simulink model "JAndrews_Test"  (R2019b)
settings: Solver=VariableStepAuto  StartTime=0.0  StopTime=10.0  RelTol=1e-3
settings Model: Creator=ng21251  LastModifiedBy=ng21251

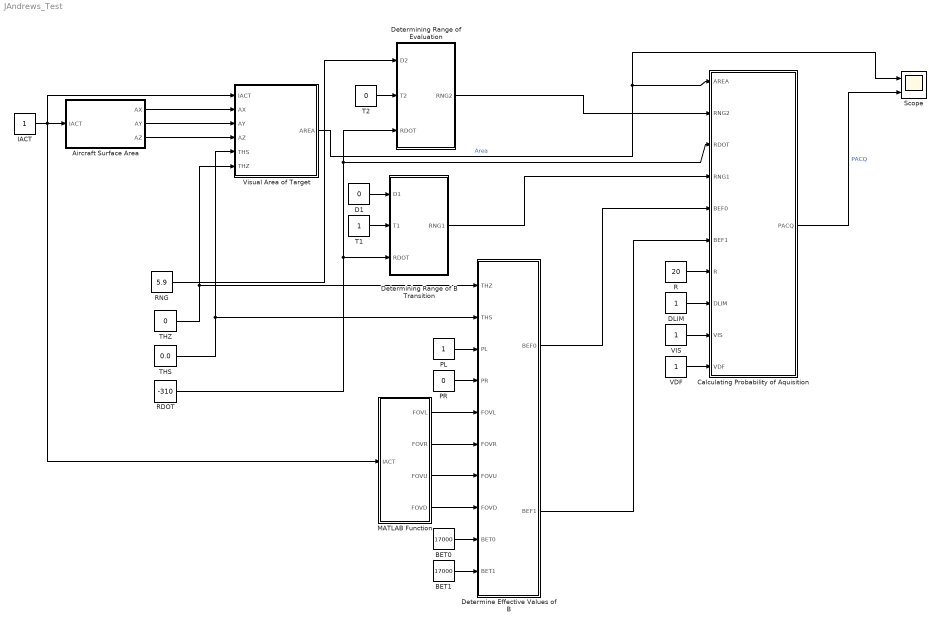
== system JAndrews_Test ==
  Aircraft Surface Area : MATLAB Function  TreatAsAtomicUnit=on
  BET0 : Constant  Value=17000
  BET1 : Constant  Value=17000
  Calculating Probability of Aquisition : MATLAB Function  TreatAsAtomicUnit=on
  D1 : Constant  Value=0
  DLIM : Constant
  Determine Effective Values of B : MATLAB Function  TreatAsAtomicUnit=on
  Determining Range of B Transition : MATLAB Function  TreatAsAtomicUnit=on
  Determining Range of Evaluation : MATLAB Function  TreatAsAtomicUnit=on
  "IACT " : Constant
  MATLAB Function : MATLAB Function  TreatAsAtomicUnit=on
  PL : Constant
  PR : Constant  Value=0
  R : Constant  Value=20
  "RDOT " : Constant  Value=-310
  "RNG " : Constant  Value=5.9
  Scope : Scope  NumInputPorts=2
  T1 : Constant
  T2 : Constant  Value=0
  THS : Constant  Value=0.0
  THZ : Constant  Value=0
  "VDF " : Constant
  VIS : Constant
  Visual Area of Target : MATLAB Function  TreatAsAtomicUnit=on
  wires:
  MATLAB Function/2(FOVR) -> Determine Effective Values of B/6(FOVR)
  Determining Range of Evaluation/1(RNG2) -> Calculating Probability of Aquisition/2(RNG2)
  "IACT "/1 -> Visual Area of Target/1(IACT), MATLAB Function/1(IACT), Aircraft Surface Area/1(IACT)
  Determine Effective Values of B/1(BEF0) -> Calculating Probability of Aquisition/5(BEF0)
  "RNG "/1 -> Determining Range of Evaluation/1(D2)
  Visual Area of Target/1(AREA) -> Scope/1, Calculating Probability of Aquisition/1(AREA)  "Area"
  R/1 -> Calculating Probability of Aquisition/7(R)
  DLIM/1 -> Calculating Probability of Aquisition/8(DLIM)
  Determine Effective Values of B/2(BEF1) -> Calculating Probability of Aquisition/6(BEF1)
  Aircraft Surface Area/2(AY) -> Visual Area of Target/3(AY)
  T2/1 -> Determining Range of Evaluation/2(T2)
  D1/1 -> Determining Range of B Transition/1(D1)
  Aircraft Surface Area/1(AX) -> Visual Area of Target/2(AX)
  Determining Range of B Transition/1(RNG1) -> Calculating Probability of Aquisition/4(RNG1)
  PL/1 -> Determine Effective Values of B/3(PL)
  MATLAB Function/1(FOVL) -> Determine Effective Values of B/5(FOVL)
  Aircraft Surface Area/3(AZ) -> Visual Area of Target/4(AZ)
  THS/1 -> Determine Effective Values of B/2(THS), Visual Area of Target/5(THS)
  PR/1 -> Determine Effective Values of B/4(PR)
  T1/1 -> Determining Range of B Transition/2(T1)
  "RDOT "/1 -> Determining Range of B Transition/3(RDOT), Determining Range of Evaluation/3(RDOT), Calculating Probability of Aquisition/3(RDOT)
  Calculating Probability of Aquisition/1(PACQ) -> Scope/2  "PACQ"
  THZ/1 -> Determine Effective Values of B/1(THZ), Visual Area of Target/6(THZ)
  BET0/1 -> Determine Effective Values of B/9(BET0)
  BET1/1 -> Determine Effective Values of B/10(BET1)
  MATLAB Function/4(FOVD) -> Determine Effective Values of B/8(FOVD)
  MATLAB Function/3(FOVU) -> Determine Effective Values of B/7(FOVU)
  "VDF "/1 -> Calculating Probability of Aquisition/10(VDF)
  VIS/1 -> Calculating Probability of Aquisition/9(VIS)

== matlab function JAndrews_Test/Calculating Probability of Aquisition ==
  data: AREA input; PACQ output; RNG2 input; RDOT input; RNG1 input; BEF0 input; BEF1 input; R input; DLIM input; VIS input; VDF input
function PACQ = JAndrews_Mod_7(AREA, RNG2, RDOT, RNG1, BEF0, BEF1, R, DLIM, VIS, VDF)
% Input variable defintions
% No, symbol, name, value, definition
% 7.  R,  R,    20. nmi,                  visual range
% 8.  d,  DLIM, 1 arc-min,                Resolution limit of human eye.
% 17. r., RDOT, 380 kt*,                  Range rate of target aircraft
% 21. A,  AREA, 35 sq.ft.*,               Final visual area of target.
% 24. R1, RNG1, 3.78 nmi*,                Range at which B transition occurs.
% 25. R2, RNG2, 1.27 nmi*,                Range at which PACQ is evaluated.
% 26. B0, BEF0, 17000* per steradian-sec, Effective value of B before transition.
% 27. B1, BEF1, 17000* per steradian-sec, Effective value of B after transition.
% 28. P, PACQ,  -                         Probability of visual aquisition
% *=value that is computed when all 16 input variables have nominal value.
 
 
% 4.2.7 Module 7: timputing the Wmulative Probability of kquiaition
% M
% Module 7 ia the final module that actually computes the probability of
% visual acquisition, PACQ. It requires 8 inputa aa ahom in Fig. 4.1.
% Module 7 aaaumes that the acquisition rate drops immediately to zero when
% the target ia beyond a range, RLIM, corresponding to the resolution limit of
% the human eye. RLIM ia defined aa follows: First, DL~, WA, and RDOT are
% used to compute the range at which the solid angle subtended by the target
% equals that of a circle with diameter DL~. This range ia given by the
% formula
% 1.1284*SQRT(AREA)/DLIM
% where DL~ ia in radiana. Then, if this range is greater than R, the visual
% range, it is reduced to R. The net result ia
% RLIM = ndnimum [1.1284*SQRT(A~A)/DLIM, R]
% A more aophieticated model for MIM could be constructed, but in meet
% analyaea, only a tiny fraction of the opportunity for visual acquieition
% occurs before the target ie well within visual range and well above the
% resolution threshold. Wnce, the detaile of the model in this regard are
% normally of little consequence.
% Note that if RLIM ia less than RNGl, then % till already have
% transitioned to BET1 before the target is close enough to be seen. b this
% caae, the value of BETO has no affect upon the calculation.
 
%Range limit = the minimum of either the human eye distinguishing target size or visual range
RLIM = min([ 1.1284 * (AREA)^0.5 / DLIM, R]);

%if the eval range is beyond these two - cannot detect
if RNG2 > RLIM 
    PACQ=0;
    
else
    
%else
    rng3=intcalcforce(AREA,RNG2,RDOT);
    pacq_3= BEF0*(rng3)*VIS*VDF;
    PACQ=1.0-exp(-pacq_3);

end


function x_e = intcalcforce(A,B,C)
T2=0:0.0001:1;

tmp=(A./(B+C*T2).^2).* exp(-2.996 * (B+C*T2));
x_e=sum(tmp*0.0001)*((numel(T2)-1)/numel(T2));

== matlab function JAndrews_Test/Visual Area of Target ==
  data: IACT input; AX input; AREA output; AY input; AZ input; THS input; THZ input
function AREA = JAndrews_Mod_3(IACT,AX, AY, AZ, THS, THZ)
% Input variable defintions
% No, symbol, name, value, definition
% 18. Ax, AX,   35 sq.ft.*,               Head-on visual area of target.
% 19. Ay, AY,   85 sq.ft.*,               Broadside visual area of target.
% 20. Az, AZ,   260 sq.ft.*,              Topside visual area of target.
% 21. A,  AREA, 35 sq.ft.*,               Final visual area of target.
% 22. 0T, TH1,  0 deg*,                   Bearing of target aircraft as seen from subject aircraft.
% 23. 0S, TH2,  0 deg*,                   Bearing of subject aircraft as seen from target aircraft.
% 24. R1, RNG1, 3.78 nmi*,                Range at which B transition occurs.
% 25. R2, RNG2, 1.27 nmi*,                Range at which PACQ is evaluated.
% 26. B0, BEF0, 17000* per steradian-sec, Effective value of B before transition.
% 27. B1, BEF1, 17000* per steradian-sec, Effective value of B after transition.
% 28. P, PACQ,  -                         Probability of visual aquisition
% *=value that is computed when all 16 input variables have nominal value.



%%-------MODULE 3---------
% 4.2.3 Module 3: Computing the Visual Area of the Target
% The visual area of the target ie computed by projecting the principal
% visual areas AX and AY onto a plane that is normal to the linemf-sfght
% between the two aircraft. ~is plane is at an angle ~ with respect to the
% Y-Z plane for the target aircraft. h approximate correction for shielding ie
% applied by assudng that the actual visual area is the largest of the
% projectione of M and AY plus one+hird of the smallest projection (see
% Mference 2). ~is approximation is errorless when the aircraft ie viewed
% along one of the principal axas. Because Mdule 3 assumes that the
% line-f =ight lies tithin the X-Y plane, the topside area, AZ, ie not allowed
% to centribute to the target visual area. This ia normally a good assumption,
% but can result in underestimation of the visual area if the pitch angle of the
% aircraft is large. U is defined in the module to allow for future exteneion
% of the software.



if IACT>7
% aclist=[...
% 'a10 ';'a109';'a306';'a310';'a318';'a319';'a320';'a321';'a332';'a333';'a342';
% 'a343';'a345';'a346';'a6  ';'aa5 ';'aest';'as32';'as50';'as55';'as65';'astr';'at72';
% 'b06 ';'b190';'b2  ';'b200';'b206';'b222';'b350';'b400';'b412';'b427';'b461';'b462';
% 'b52 ';'b703';'b712';'b721';'b722';'b731';'b732';'b733';'b734';'b735';'b737';'b738';
% 'b743';'b744';'b752';'b753';'b762';'b763';'b772';'b773';'be18';'be20';'be35';'be40';
% 'be50';'be56';'be58';'be60';'be70';'be90';'be99';'bk17';'c130';'c141';'c152';'c17 ';
% 'c172';'c177';'c182';'c185';'c206';'c208';'c210';'c212';'c310';'c402';'c5  ';'c500';
% 'c680';'c750';'cl60';'col3';'crj1';'crj2';'crj7';'crj9';'d328';'dc10';'dc3 ';'dc91';
% 'dc93';'dc95';'dh8a';'dh8b';'dh8c';'dh8d';'e110';'e121';'e135';'e145';'e170';'e190';
% 'e2  ';'e45x';'e767';'ec20';'ec35';'ec45';'f100';'f14 ';'f15 ';'f16 ';'f18 ';'f22 ';
% 'f2th';'f900';'fa10';'fa50';'galx';'glex';'glf4';'glf5';'h25b';'h47 ';'h500';'h53s';
% 'h60 ';'h64 ';'huco';'js31';'k35e';'k35r';'lj31';'lj35';'lj45';'lj60';'m20p';'md11';
% 'md60';'md81';'md82';'md83';'md88';'mi2 ';'mi24';'mi28';'mu2 ';'p28a';'p3  ';'pa11';
% 'pa22';'pa23';'pa31';'pa32';'pa44';'pa46';'pc12';'r22 ';'rq1 ';'rq4a';'s360';'s65c';
% 'sf34';'sh33';'sr20';'sr71';'sw4 ';'u2  ';'uh1 ';'v22 ';'vc10';'ww24'];
AREA_S=[     0   -90   414
    15   -90   591
    30   -90   601
    45   -90   588
    60   -90   591
    75   -90   589
    90   -90   414
   105   -90   596
   120   -90   602
   135   -90   588
   150   -90   591
   165   -90   591
   180   -90   416
   195   -90   591
   210   -90   601
   225   -90   588
   240   -90   596
   255   -90   589
   270   -90   416
   285   -90   601
   300   -90   601
   315   -90   589
   330   -90   591
   345   -90   589
   360   -90   414
     0   -75   392
    15   -75   392
    30   -75   388
    45   -75   407
    60   -75   413
    75   -75   566
    90   -75   485
   105   -75   444
   120   -75   444
   135   -75   434
   150   -75   469
   165   -75   546
   180   -75   546
   195   -75   543
   210   -75   428
   225   -75   461
   240   -75   472
   255   -75   472
   270   -75   468
   285   -75   478
   300   -75   407
   315   -75   401
   330   -75   382
   345   -75   380
   360   -75   392
     0   -60   339
    15   -60   360
    30   -60   430
    45   -60   441
    60   -60   481
    75   -60   540
    90   -60   540
   105   -60   463
   120   -60   448
   135   -60   517
   150   -60   511
   165   -60   506
   180   -60   499
   195   -60   494
   210   -60   500
   225   -60   427
   240   -60   450
   255   -60   440
   270   -60   461
   285   -60   535
   300   -60   481
   315   -60   441
   330   -60   426
   345   -60   358
   360   -60   339
     0   -45   271
    15   -45   353
    30   -45   374
    45   -45   392
    60   -45   387
    75   -45   359
    90   -45   356
   105   -45   376
   120   -45   431
   135   -45   437
   150   -45   431
   165   -45   412
   180   -45   407
   195   -45   416
   210   -45   414
   225   -45   442
   240   -45   375
   255   -45   386
   270   -45   329
   285   -45   344
   300   -45   336
   315   -45   380
   330   -45   376
   345   -45   352
   360   -45   271
     0   -30   333
    15   -30   345
    30   -30   349
    45   -30   366
    60   -30   348
    75   -30   292
    90   -30   312
   105   -30   290
   120   -30   356
   135   -30   343
   150   -30   327
   165   -30   327
   180   -30   297
   195   -30   323
   210   -30   337
   225   -30   345
   240   -30   357
   255   -30   300
   270   -30   294
   285   -30   280
   300   -30   336
   315   -30   363
   330   -30   357
   345   -30   344
   360   -30   333
     0   -15   229
    15   -15   247
    30   -15   259
    45   -15   243
    60   -15   315
    75   -15   305
    90   -15   275
   105   -15   314
   120   -15   290
   135   -15   253
   150   -15   216
   165   -15   229
   180   -15   189
   195   -15   250
   210   -15   216
   225   -15   250
   240   -15   289
   255   -15   314
   270   -15   278
   285   -15   276
   300   -15   314
   315   -15   237
   330   -15   244
   345   -15   248
   360   -15   229
     0     0   125
    15     0   180
    30     0   206
    45     0   208
    60     0   264
    75     0   289
    90     0   288
   105     0   280
   120     0   265
   135     0   208
   150     0   202
   165     0   182
   180     0   125
   195     0   180
   210     0   206
   225     0   208
   240     0   264
   255     0   289
   270     0   288
   285     0   280
   300     0   265
   315     0   208
   330     0   202
   345     0   182
   360     0   125
     0    15   192
    15    15   250
    30    15   216
    45    15   250
    60    15   289
    75    15   314
    90    15   278
   105    15   276
   120    15   314
   135    15   237
   150    15   244
   165    15   248
   180    15   229
   195    15   247
   210    15   259
   225    15   243
   240    15   315
   255    15   305
   270    15   275
   285    15   314
   300    15   290
   315    15   253
   330    15   216
   345    15   229
   360    15   192
     0    30   299
    15    30   323
    30    30   337
    45    30   345
    60    30   357
    75    30   300
    90    30   294
   105    30   280
   120    30   336
   135    30   363
   150    30   357
   165    30   344
   180    30   333
   195    30   345
   210    30   349
   225    30   366
   240    30   348
   255    30   292
   270    30   312
   285    30   290
   300    30   356
   315    30   343
   330    30   327
   345    30   327
   360    30   299
     0    45   405
    15    45   416
    30    45   414
    45    45   442
    60    45   375
    75    45   386
    90    45   329
   105    45   344
   120    45   336
   135    45   380
   150    45   376
   165    45   352
   180    45   271
   195    45   353
   210    45   374
   225    45   392
   240    45   387
   255    45   359
   270    45   356
   285    45   376
   300    45   431
   315    45   437
   330    45   431
   345    45   412
   360    45   405
     0    60   496
    15    60   494
    30    60   500
    45    60   427
    60    60   450
    75    60   440
    90    60   461
   105    60   535
   120    60   481
   135    60   441
   150    60   426
   165    60   358
   180    60   339
   195    60   360
   210    60   430
   225    60   441
   240    60   481
   255    60   540
   270    60   540
   285    60   463
   300    60   448
   315    60   517
   330    60   511
   345    60   506
   360    60   496
     0    75   546
    15    75   543
    30    75   428
    45    75   461
    60    75   472
    75    75   472
    90    75   468
   105    75   478
   120    75   407
   135    75   401
   150    75   382
   165    75   375
   180    75   396
   195    75   399
   210    75   388
   225    75   407
   240    75   413
   255    75   566
   270    75   485
   285    75   444
   300    75   444
   315    75   434
   330    75   469
   345    75   546
   360    75   546
     0    90   414
    15    90   596
    30    90   601
    45    90   588
    60    90   596
    75    90   591
    90    90   416
   105    90   591
   120    90   601
   135    90   589
   150    90   596
   165    90   591
   180    90   414
   195    90   596
   210    90   601
   225    90   589
   240    90   591
   255    90   589
   270    90   414
   285    90   601
   300    90   602
   315    90   589
   330    90   596
   345    90   589
   360    90   414];

    THSdiff=abs(AREA_S(:,1)-THS);
    THZdiff=abs(AREA_S(:,2)-THZ);
    mTHS=min(THSdiff);
    mTHZ=min(THZdiff);
    
    %find the closest angle combination
    indx=ismember(THSdiff,mTHS)&ismember(THZdiff,mTHZ);
    
    %make a list of indicies
    %find the incidices that are the closest
    %take the first instance only
    indxnum=1:numel(indx);
    indxnum=indxnum(indx>0);
    indxnum=indxnum(1);
    
    %area = first smallest index - convert to nm^2
    AREA=AREA_S(indxnum,3)/6076.115486;
    
    
else

XArea = abs(cos(deg2rad(THS))) * abs(cos(deg2rad(THZ))) * AX;
YArea = abs(sin(deg2rad(THS))) * abs(cos(deg2rad(THZ))) * AY;

ZArea = abs(sin(deg2rad(THZ))) * AZ;



AREA = XArea + YArea + ZArea;
AREA=AREA/6076.115486;
end

== matlab function JAndrews_Test/Aircraft Surface Area ==
  data: IACT input; AX output; AY output; AZ output
function [AX, AY, AZ] = JAndrews_Mod_1(IACT)

% Input variable defintions
% No, symbol, name, value, definition
% 1.  - , BET0, 17000 per steradian-sec,  single pilot B values before transition
% 2.  - , BET1, 17000 per steradian-sec,  Single-pilot B value after transition
% 3.  t1, T1,   180 sec,                  modified tau time for B transition (time to closest approach)
% 4.  t2, T2,   12 sec,                   modified tau time for evaluation of PACQ (time to closest approach)
% 5.  D1, D1,   0. nmi,                   modified tau range parameter for B transition.
% 6.  D2, D2,   0. nmi,                   modified tau range parameter for PACQ evaluation
% 7.  R,  R,    20. nmi,                  visual range
% 8.  d,  DLIM, 1 arc-min,                Resolution limit of human eye.
% 9.  V1, VSUB1,180 kt,                   airspeed of subject aircraft.
% 10. V2, VSUB2,130 kt,                   airspeed of target aircraft.
% 11. - , IACT, 1,                        aircraft type for target aircraft (see table)
% 12. X,  XANG, 180. deg,                 Crossing angle (relative heading)
% 13. PL, PL,   1.0,                      Search intensity for pilot in left seat (0 = no pilot, 1 = normal search)
% 14. PR, PR,   1.0,                      Search intensity for pilot in right seat (0 = no pilot, 1 = normal search)
% 15. FL, FOVL, -120 degrees              Field-of-view cutoff on left side for searching pilot in left seat (measured positive clockwise from straight ahead). 
% 16. FR, FOVR, -90 degrees               Field-of-view cutoff on left side for searching pilot in right seat (measured positive clockwise from straight ahead). 
% 17. r., RDOT, 380 kt*,                  Range rate of target aircraft
% 18. Ax, AX,   35 sq.ft.*,               Head-on visual area of target.
% 19. Ay, AY,   85 sq.ft.*,               Broadside visual area of target.
% 20. Az, AZ,   260 sq.ft.*,              Topside visual area of target.
% 21. A,  AREA, 35 sq.ft.*,               Final visual area of target.
% 22. 0T, TH1,  0 deg*,                   Bearing of target aircraft as seen from subject aircraft.
% 23. 0S, TH2,  0 deg*,                   Bearing of subject aircraft as seen from target aircraft.
% 24. R1, RNG1, 3.78 nmi*,                Range at which B transition occurs.
% 25. R2, RNG2, 1.27 nmi*,                Range at which PACQ is evaluated.
% 26. B0, BEF0, 17000* per steradian-sec, Effective value of B before transition.
% 27. B1, BEF1, 17000* per steradian-sec, Effective value of B after transition.
% 28. P, PACQ,  -                         Probability of visual aquisition
% *=value that is computed when all 16 input variables have nominal value.

% Parameters for encounter
% IACT
% V1
% V2
% T1
% D1
% R
% PL, PR, DLIM, FOVL, FOVR, BET0, XANG, BET1, T2, D2
%% ------------------ MODULE 1 ---------------------------------
%Aircarft types used - structure
tmpstruct=struct('IACT',0,'ACTYPE','                    ','NAME','                    ','AX',0,'AY',0,'AZ',0);
AC_Struct=[tmpstruct;tmpstruct;tmpstruct;tmpstruct;tmpstruct;tmpstruct;tmpstruct];
for it=1:7

     AC_Struct(1).IACT=1;
           AC_Struct(1).ACTYPE=['Piper PA-28',blanks(20-numel('Piper PA-28'))];
            AC_Struct(1).NAME=['PA28',blanks(20-numel('PA28'))];
            AC_Struct(1).AX=35;
            AC_Struct(1).AY=85;
            AC_Struct(1).AZ=260;

    AC_Struct(2).IACT=2;
            AC_Struct(2).ACTYPE=['Seeing 727',blanks(20-numel('Seeing 727'))];
            AC_Struct(2).NAME=['B727',blanks(20-numel('B727'))];
            AC_Struct(2).AX=400;
            AC_Struct(2).AY=1900;
            AC_Struct(2).AZ=3100;

    AC_Struct(3).IACT=3;
            AC_Struct(3).ACTYPE=['Boeing 747',blanks(20-numel('Boeing 747'))];
            AC_Struct(3).NAME=['B747',blanks(20-numel('B747'))];
            AC_Struct(3).AX=1200;
            AC_Struct(3).AY=5700;
            AC_Struct(3).AZ=9300;

    AC_Struct(4).IACT=4;
            AC_Struct(4).ACTYPE=['MDonnell-Douglas DC9',blanks(20-numel('MDonnell-Douglas DC9'))];
            AC_Struct(4).NAME=['DC9',blanks(20-numel('DC9'))];
            AC_Struct(4).AX=300;
            AC_Struct(4).AY=1425;
            AC_Struct(4).AZ=2325;

      AC_Struct(5).IACT=5;
          AC_Struct(5).ACTYPE=['Ceesna 421',blanks(20-numel('Ceesna 421'))];
            AC_Struct(5).NAME=['C421',blanks(20-numel('C421'))];
            AC_Struct(5).AX=81;
            AC_Struct(5).AY=171;
            AC_Struct(5).AZ=417;

    AC_Struct(6).IACT=6;
            AC_Struct(6).ACTYPE=['U-21 (fing fir)',blanks(20-numel('U-21 (fing fir)'))];
            AC_Struct(6).NAME=['U21',blanks(20-numel('U21'))];
            AC_Struct(6).AX=127;
            AC_Struct(6).AY=267;
            AC_Struct(6).AZ=600;
 
    AC_Struct(7).IACT=7;
            AC_Struct(7).ACTYPE=['F-18',blanks(20-numel('F-18'))];
            AC_Struct(7).NAME=['F18',blanks(20-numel('F18'))];
            AC_Struct(7).AX=50;
            AC_Struct(7).AY=280;
            AC_Struct(7).AZ=540;
end
%Return values for AC of interest as square nautical miles
AX = AC_Struct(IACT).AX;
AY = AC_Struct(IACT).AY;
AZ = AC_Struct(IACT).AZ;

== matlab function JAndrews_Test/Determining Range of B Transition ==
  data: D1 input; RNG1 output; T1 input; RDOT input
function RNG1 = JAndrews_Mod_6(D1,T1,RDOT)
% Input variable defintions
% No, symbol, name, value, definition
% 3.  t1, T1,   180 sec,                  modified tau time for B transition (time to closest approach)
% 5.  D1, D1,   0. nmi,                   modified tau range parameter for B transition.
% 17. r., RDOT, 380 kt*,                  Range rate of target aircraft
% 24. R1, RNG1, 3.78 nmi*,                Range at which B transition occurs.
% *=value that is computed when all 16 input variables have nominal value.

%% Modeule 6 -
% 4.2.6 Wdule 6: Determining the tinge of 8 Transition
% In a particular scenario, the nominal value of 6 for a single pilot mey
% be alterad by an event such as the receipt of a traffic advieory.SEE1 allowa
% the notinal single~ilot value of 6 to transition from one value to another at
% a predefined point during the encounter. The initial value of 6 is BETO.
% After the transition, the value of B fa BET1 (see Fig. 4.6). The range at
% which trzaaition occurs ia NG1. It is computed using a modified tau
% criterion involving the two input parameter DI and RI:
% 
% RNG1 = D1 - ROOT*T1
% 
% The transition occurs when the target is T1 secondefrom reaching a
% range D1. Note that if TI=O, then a simple range criterion results. H D1=O,
% then a simple time-to-collision criterion reeulta.
% If the application of interest does not require a transition, the
% transition ie easily avoided by setting BET1 equal to BETO. The eettings of
% D1 and T1 then have no effect upon the computations (becauae the valuee of 8
% are unchanged by reaching the transition point).

%RNG1 = D1 (0 nmi) - RDOT (kts) * T1 (seconds)

RNG1 = D1 - RDOT * T1;

== matlab function JAndrews_Test/Determining Range of Evaluation ==
  data: D2 input; RNG2 output; T2 input; RDOT input
function RNG2 = JAndrews_Mod_5(D2, T2, RDOT)
% Input variable defintions
% No, symbol, name, value, definition
% 4.  t2, T2,   12 sec,                   modified tau time for evaluation of PACQ (time to closest approach)
% 6.  D2, D2,   0. nmi,                   modified tau range parameter for PACQ evaluation
% 17. r., RDOT, 380 kt*,                  Range rate of target aircraft
% 25. R2, RNG2, 1.27 nmi*,                Range at which PACQ is evaluated.
% *=value that is computed when all 16 input variables have nominal value.

%%  4.2.5 Module 5: Determining the ~nge of Evaluation
% The cumulative probability of visual acquisition, PACQ, depends upon the
% range, MG2, at which PACQ ia to be evaluated: Often it ia desirable to aet
% this ranga to the latest point at which sufficient time exists for evasive
% action. Then PACQ till repreeent tha probability of visual acquisition with
% aufficient lead time for avoidanca.
% RNG2 ie computed using a modified tau criterion based upon two input
% parameter D2 and U:
% ~G2 = D2 - ~OT*T2
% From thie equation it can be seen that SNG2 ie reached when tbe target
% ia T2 seconds from reaching a range of D2. with this formulation, WG2 can
% be deterdned as either a constant range, a constant time-to-collision, or a
% modified tau criterion. For example, if T2=0, then the equation yields a
% simple range critaria for which PACQ is evaluated at range D2. If D2=0,
% then a simple time critaria results in which PACQ La evaluated when T2
% secoada remain befora collision. If neither T2 nor D2 are zero, then a
% modified tau criterion results.

%RNG2 = D2 (0 nmi) - RDOT (kts) * T2 (12 seconds)

RNG2 = D2 - RDOT * T2;

== matlab function JAndrews_Test/Determine Effective Values of B ==
  data: THZ input; BEF0 output; THS input; PL input; PR input; FOVL input; FOVR input; FOVU input; FOVD input; BET0 input; BET1 input; BEF1 output
function [BEF0, BEF1] = JAndrews_Mod_4(THZ, THS, PL, PR, FOVL, FOVR, FOVU, FOVD, BET0, BET1)
% Input variable defintions
% No, symbol, name, value, definition
% 1.  - , BET0, 17000 per steradian-sec,  single pilot B values before transition
% 2.  - , BET1, 17000 per steradian-sec,  Single-pilot B value after transition
% 13. PL, PL,   1.0,                      Search intensity for pilot in left seat (0 = no pilot, 1 = normal search)
% 14. PR, PR,   1.0,                      Search intensity for pilot in right seat (0 = no pilot, 1 = normal search)
% 15. FL, FOVL, -120 degrees              Field-of-view cutoff on left side for searching pilot in left seat (measured positive clockwise from straight ahead). 
% 16. FR, FOVR, 90 degrees               Field-of-view cutoff on left side for searching pilot in right seat (measured positive clockwise from straight ahead). 
% 23. 0S, TH2(THT),  0 deg*,              Bearing of subject aircraft as seen from target aircraft.
% 26. B0, BEF0, 17000* per steradian-sec, Effective value of B before transition.
% 27. B1, BEF1, 17000* per steradian-sec, Effective value of B after transition.
% 28. P, PACQ,  -                         Probability of visual aquisition
% *=value that is computed when all 16 input variables have nominal value.

%% 4.2.4 Module 4: Wtermining the Effective Values of 6
% Module 4 examinee cockpit visibility and crew complement in order to
% deterfine their effect upon search effectiveness. It does eo by taking the
% notinal single~ilot B values and ebng them to produce effective B
% values. For a single pilot devoting normal effort to visual search, the
% value of S before and afterthetransitionevent(eee4.2.6)are represented
% by parameter BETO and BET1. Module 4 computes two corresponding effective
% 8 values, BEFO and BEF1, by e-rig the 8 values for each pilot who ie able to
% contribute to visual search.
% 
% The fieldmf~iew of the cockpit is deter~ned by the variables FOW and
% FOPS (ace Fig. 4.5). It ia aesumed that the cockpit visibility ia symmetric
% and that there is no cut~ff in elevation (normally true for targeta on
% collision courses). Tfienthe target ~a outside the field-f -iew, the
% effective 6 velue is set to zero.
% By setting FL and ~, the user specifies the number of pilots that
% contribute to search for both left and right visibility limite. Normally PL
% and ~ are efther sero (no pilot in the seat) or unity (single pilot in seat
% and eearching normally). It is possible to use a value between O and 1 to
% represent a pilot who is preeent, but ia devoting less than the normal amount
% of time to visual search. Or a value greater than 1 can be used to represent
% search by an additional crew member.
% 
% For the nominal input values given in Table 3.1, it ia assumed that a
% single pilot is searching from the left seat of the aircraft (PL=l.O, pR=O.O).
% For the notinal values of croesing angle (WG-180 degrees), tha intruder is
% always within the field of view. Thus for the nominal input values, BEFO=BETO
% and BEF1=BET1.

%% CHECK FOR FOV L/R PILOT

%THS is now between -180 and 180;
while THS<-180
    THS=THS+180;
end
while THS>180
    THS=THS-180;
end
    
%ensure THZ is between +/-90
while THZ<-90
    THZ=THZ+90;
end
while THZ>90
    THZ=THZ-90;
end

% if left pilot present
PL_FOV = 0;
if PL
    
    %check if intruder w/in field of view
    if THS >= FOVL && THS <= FOVR &&...  %target is w/in L/R LOS
            ( (THZ >= FOVD && THZ <= FOVU) ||... %THZ is -90 to +90
            (THZ > FOVU && THZ >= FOVD + 360 && THZ < 360) ) %THZ is >270
        
            PL_FOV = 1;
        
    end
else
    PL_FOV = 0;
end

%check if right pilot present
PR_FOV=0;
if PR 
        if THS >= -FOVR && THS <= -FOVL &&...  %target is w/in L/R LOS
            ( (THZ >= FOVD && THZ <= FOVU) ||... %THZ is -90 to +90
            (THZ > FOVU && THZ >= FOVD + 360 && THZ < 360) ) %THZ is >270
        
            PR_FOV = 1;
        end
else
    PR_FOV=0;
end
        
        
%set BETs = BEFs
BEF0 = BET0 * PL_FOV + BET0 * PR_FOV;
BEF1 = BET1 * PL_FOV + BET1 * PR_FOV;

== matlab function JAndrews_Test/MATLAB Function ==
  data: IACT input; FOVL output; FOVR output; FOVU output; FOVD output
 function [FOVL, FOVR, FOVU, FOVD] = JAndrews_Mod_8  (IACT)

%field of view values derived from 
 
%Aircarft types used - structure
tmpstruct=struct('IACT',0,'ACTYPE','                    ','NAME','                    ','FOVL',0,'FOVR',0,'FOVU',0,'FOVD',0);
AC_Int_Struct=[tmpstruct;tmpstruct;tmpstruct;tmpstruct;tmpstruct;tmpstruct;tmpstruct];
for it=1:7

     AC_Int_Struct(1).IACT=1;  %one engine prop
           AC_Int_Struct(1).ACTYPE=['Piper PA-28',blanks(20-numel('Piper PA-28'))];
            AC_Int_Struct(1).NAME=['PA28',blanks(20-numel('PA28'))];
            AC_Int_Struct(1).FOVL=-120;
            AC_Int_Struct(1).FOVR=80;
            AC_Int_Struct(1).FOVU=15;
            AC_Int_Struct(1).FOVD=-10;

    AC_Int_Struct(2).IACT=2; %three jets on tail
            AC_Int_Struct(2).ACTYPE=['Seeing 727',blanks(20-numel('Seeing 727'))];
            AC_Int_Struct(2).NAME=['B727',blanks(20-numel('B727'))];
            AC_Int_Struct(2).FOVL=-120;
            AC_Int_Struct(2).FOVR=80;
            AC_Int_Struct(2).FOVU=15;
            AC_Int_Struct(2).FOVD=-10;

    AC_Int_Struct(3).IACT=3;  %4 engine jet
            AC_Int_Struct(3).ACTYPE=['Boeing 747',blanks(20-numel('Boeing 747'))];
            AC_Int_Struct(3).NAME=['B747',blanks(20-numel('B747'))];
            AC_Int_Struct(3).FOVL=-120;
            AC_Int_Struct(3).FOVR=80;
            AC_Int_Struct(3).FOVU=15;
            AC_Int_Struct(3).FOVD=-10;

    AC_Int_Struct(4).IACT=4;  %baby jet - 2 engines on tail
            AC_Int_Struct(4).ACTYPE=['MDonnell-Douglas DC9',blanks(20-numel('MDonnell-Douglas DC9'))];
            AC_Int_Struct(4).NAME=['DC9',blanks(20-numel('DC9'))];
            AC_Int_Struct(4).FOVL=-120;
            AC_Int_Struct(4).FOVR=80;
            AC_Int_Struct(4).FOVU=15;
            AC_Int_Struct(4).FOVD=-10;

      AC_Int_Struct(5).IACT=5;  %2 engine prop 
          AC_Int_Struct(5).ACTYPE=['Ceesna 421',blanks(20-numel('Ceesna 421'))];
            AC_Int_Struct(5).NAME=['C421',blanks(20-numel('C421'))];
            AC_Int_Struct(5).FOVL=-120;
            AC_Int_Struct(5).FOVR=80;
            AC_Int_Struct(5).FOVU=15;
            AC_Int_Struct(5).FOVD=-10;

    AC_Int_Struct(6).IACT=6; %multi engine prop
            AC_Int_Struct(6).ACTYPE=['U-21 (fing fir)',blanks(20-numel('U-21 (fing fir)'))];
            AC_Int_Struct(6).NAME=['U21',blanks(20-numel('U21'))];
            AC_Int_Struct(6).FOVL=-120;
            AC_Int_Struct(6).FOVR=80;
            AC_Int_Struct(6).FOVU=15;
            AC_Int_Struct(6).FOVD=-10;
 
    AC_Int_Struct(7).IACT=7; %fighter jet
            AC_Int_Struct(7).ACTYPE=['F-18',blanks(20-numel('F-18'))];
            AC_Int_Struct(7).NAME=['F18',blanks(20-numel('F18'))];
            AC_Int_Struct(6).FOVL=-120;
            AC_Int_Struct(6).FOVR=80;
            AC_Int_Struct(6).FOVU=15;
            AC_Int_Struct(6).FOVD=-10;
end

%Return values for AC of interest
FOVL = AC_Int_Struct(IACT).FOVL;
FOVR = AC_Int_Struct(IACT).FOVR;
FOVU = AC_Int_Struct(IACT).FOVU;
FOVD = AC_Int_Struct(IACT).FOVD;
